simulink model "audiopitchtimeTest"  (R2018b)
settings: Solver=VariableStepAuto  StartTime=0.0  StopTime=10.0  RelTol=1e-3
undefined symbols (not defined in the file or in its folder): ana_hopSize, syn_hopSize, winLen
libraries: dspsigops x1, dspxfrm3 x1, dspswit3 x1
settings Model: Creator=AndrewSenol  LastModifiedBy=AndrewSenol

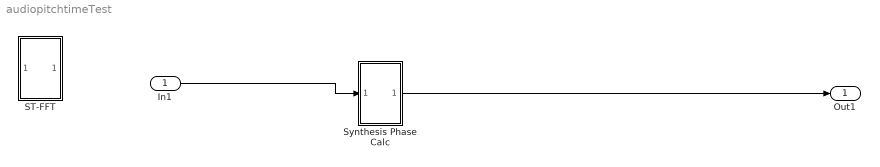
== system audiopitchtimeTest ==
  In1 : Inport
  "ST-FFT " : Subsystem
  "Synthesis Phase Calc " : Subsystem
  Out1 : Outport
  wires:
  In1/1 -> "Synthesis Phase Calc "/1(In1)
  "Synthesis Phase Calc "/1(Out1) -> Out1/1

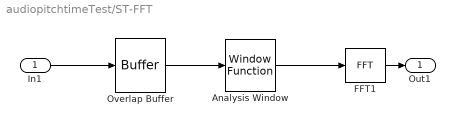
== system audiopitchtimeTest/ST-FFT  ==
  In1 : Inport
  Analysis Window : dspsigops/Window Function  winmode=Apply window to input  wintype=Hanning  sampmode=Continuous  samptime=1  N=64  Rs=50  beta=10  winsamp=Periodic  UserWindow=hamming  OptParams=off  UserParams={1.0}  dataType=double  isSigned=on  wordLen=16  udDataType=sfix(16)  fracBitsMode=Best precision  numFracBits=15  roundingMode=Floor  overflowMode=off  numSidelobes=4  sidelobeLevel=-30
      settings: SourceProductName=DSP System Toolbox  SourceProductBaseCode=DS
  FFT1 : dspxfrm3/FFT  FFTImplementation=Auto  CompMethod=Table lookup  TableOpt=NEW  TableOptActive=Speed  BitRevOrder=off  Normalize=off  InheritFFTLength=on  FFTLength=64  WrapInput=on  roundingMode=Floor  overflowMode=off  firstCoeffMode=Specify word length  firstCoeffWordLength=16  firstCoeffFracLength=15  firstCoeffDataTypeStr=fixdt(1,16)  firstCoeffLastDataTypeStr=fixdt(1,16)  accumDataTypeStr=Inherit: Same as product output  accumLastDataTypeStr=Inherit: Same as product output  outputMin=[]  outputMax=[]
  Overlap Buffer : Buffer  N=winLen  V=winLen-ana_hopSize  OutputFrames=off
  Out1 : Outport
  wires:
  In1/1 -> Overlap Buffer/1
  Analysis Window/1 -> FFT1/1
  FFT1/1 -> Out1/1
  Overlap Buffer/1 -> Analysis Window/1

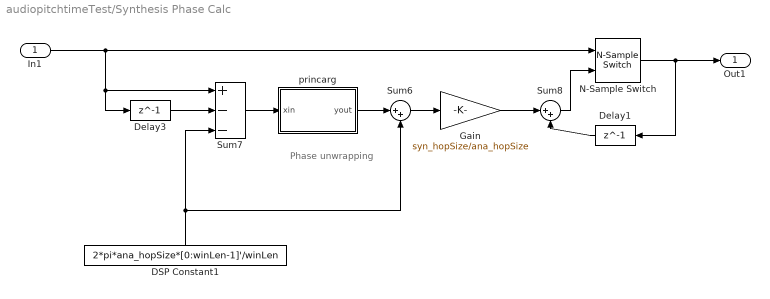
== system audiopitchtimeTest/Synthesis Phase Calc  ==
  note: Phase unwrapping
  In1 : Inport
  DSP Constant1 : Constant  Value=2*pi*ana_hopSize*[0:winLen-1]'/winLen  VectorParams1D=off  SampleTime=64/8000
  Delay1 : Delay  DelayLength=1  InitialCondition=0
  Delay3 : Delay  DelayLength=1  InitialCondition=0
  Gain : Gain  Gain=syn_hopSize/ana_hopSize  OutDataTypeStr=Inherit: Same as input  ParamDataTypeStr=Inherit: Same as input
  N-Sample Switch : dspswit3/N-Sample Switch  N=1  reset=off  TriggerType=Rising edge  Ts=-1
      settings: SourceProductName=DSP System Toolbox  SourceProductBaseCode=DS
  Sum6 : Sum  Inputs=|++  SaturateOnIntegerOverflow=on
  Sum7 : Sum  Inputs=+--  SaturateOnIntegerOverflow=on
  Sum8 : Sum  Inputs=|++  SaturateOnIntegerOverflow=on
  princarg : Subsystem
      mask Display: disp('Principal\nArgument');
  Out1 : Outport
  wires:
  Gain/1 -> Sum8/1
  Delay3/1 -> Sum7/2
  Sum6/1 -> Gain/1
  Sum8/1 -> N-Sample Switch/2
  DSP Constant1/1 -> Sum7/3, Sum6/2
  princarg/1(yout) -> Sum6/1
  In1/1 -> N-Sample Switch/1, Delay3/1, Sum7/1
  Sum7/1 -> princarg/1(xin)
  N-Sample Switch/1 -> Out1/1, Delay1/1
  Delay1/1 -> Sum8/2

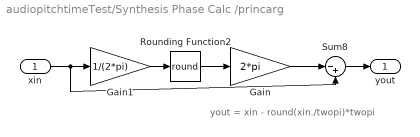
== system audiopitchtimeTest/Synthesis Phase Calc /princarg ==
  note: yout = xin - round(xin./twopi)*twopi
  xin : Inport
  Gain : Gain  Gain=2*pi  OutDataTypeStr=Inherit: Same as input  ParamDataTypeStr=Inherit: Same as input
  Gain1 : Gain  Gain=1/(2*pi)  OutDataTypeStr=Inherit: Same as input  ParamDataTypeStr=Inherit: Same as input
  Rounding Function2 : Rounding  Operator=round
  Sum8 : Sum  Inputs=|-+  SaturateOnIntegerOverflow=on
  yout : Outport
  wires:
  xin/1 -> Sum8/2, Gain1/1
  Gain1/1 -> Rounding Function2/1
  Rounding Function2/1 -> Gain/1
  Gain/1 -> Sum8/1
  Sum8/1 -> yout/1
